simulink model "Kubon_lab4_sim"  (R2020b)
settings: Solver=VariableStepAuto  StartTime=0.0  StopTime=10.0  RelTol=1e-3
values from neighbouring files (symbols this model uses):
  a0 = 7    [Kubon_lab4.m]
  a1 = 1    [Kubon_lab4.m]    (also in Kubon_lab6.m = Aw1*sqrt(2*g/H1); Kubon_lab6_test.m = Aw1*sqrt(2*g/H1); Kubon_lab7.m = Aw1*sqrt(2*g/(H1-H2)); Kubon_lab8.m = Aw1*sqrt(2*g/(H1-H2)))
  b = Cv1*Cv2    (= 308700000)    [Kubon_lab13.m]    (also in Kubon_lab4.m = 8; Kubon_lab5.m = 2*ksi(i)*w(i); Kubon_poprawa_lab5.m = 2*e(i)*w(i))
  du = 2    [Kubon_lab4.m]
  t0 = 50.0    (= 50)    [Kubon_lab10.m]    (also in Kubon_lab4.m = 5; Kubon_lab5.m = 0; Kubon_lab6.m = 5; Kubon_lab6_test.m = 0)
  u0 = 3    [Kubon_lab4.m]    (also in Kubon_lab5.m = 0; Kubon_poprawa_lab5.m = 0)
  x0 = 0    [Kubon_lab4.m]    (also in Kubon_lab5.m; Kubon_lab8.m = [h10,h20])
settings Model: Creator=pkubo  LastModifiedBy=pkubo

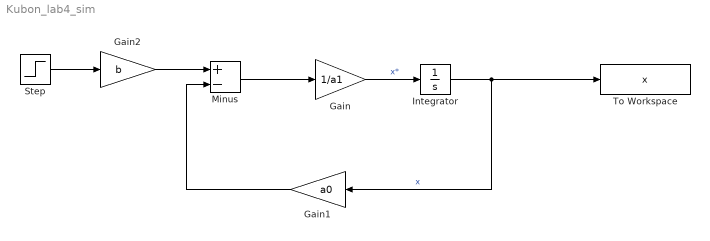
== system Kubon_lab4_sim ==
  Gain : Gain  Gain=1/a1
  Gain1 : Gain  Gain=a0
  Gain2 : Gain  Gain=b
  Integrator : Integrator  InitialCondition=x0
  Minus : Sum  Inputs=+-
  Step : Step  Time=t0  Before=u0  After=u0+du  SampleTime=0
  To Workspace : ToWorkspace  VariableName=x  SampleTime=-1
  wires:
  Minus/1 -> Gain/1
  Gain/1 -> Integrator/1  "x*"
  Integrator/1 -> Gain1/1, To Workspace/1  "x"
  Gain1/1 -> Minus/2
  Step/1 -> Gain2/1
  Gain2/1 -> Minus/1
